simulink model "Opgave1_2"  (R2017a)
settings: Solver=VariableStepAuto  StartTime=0.0  StopTime=10.0  RelTol=1e-3
values from neighbouring files (symbols this model uses):
  A = 1    [Opgave1_2_script.m]
  K1 = 10    [Opgave1_2_script.m]
  Kv = 0.5    [Opgave1_2_script.m]
  P0 = 0    [Opgave1_2_script.m]
  Qin = 2    [Opgave1_2_script.m]
settings Model: Creator=Sebastian  LastModifiedBy=Sebastian

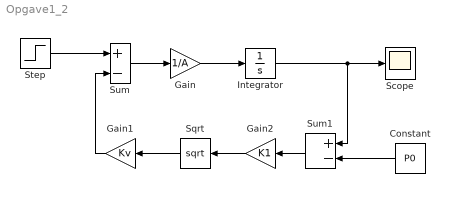
== system Opgave1_2 ==
  Constant : Constant  Value=P0
  Gain : Gain  Gain=1/A
  Gain1 : Gain  Gain=Kv
  Gain2 : Gain  Gain=K1
  Integrator : Integrator
  Scope : Scope
  Sqrt : Sqrt  SaturateOnIntegerOverflow=on
  Step : Step  After=Qin  SampleTime=0
  Sum : Sum  Inputs=+-
  Sum1 : Sum  Inputs=+-
  wires:
  Step/1 -> Sum/1
  Sum/1 -> Gain/1
  Gain/1 -> Integrator/1
  Integrator/1 -> Sum1/1, Scope/1
  Gain1/1 -> Sum/2
  Sqrt/1 -> Gain1/1
  Gain2/1 -> Sqrt/1
  Constant/1 -> Sum1/2
  Sum1/1 -> Gain2/1
